simulink model "MIL_ASW"  (R2019b)
settings: Solver=FixedStepDiscrete  StartTime=0.0  StopTime=2  FixedStep=0.001  RelTol=1e-3  EnableMultiTasking=on
model workspace (MAT data in the model file):
  AccPedlCanVal : Simulink.Signal (value not decoded)
  AccPedlVal : Simulink.Signal (value not decoded)
  BrkPedlCanVal : Simulink.Signal (value not decoded)
  BrkPedlVal : Simulink.Signal (value not decoded)
  Cal1 : Simulink.Parameter (value not decoded)
  Cal10 : Simulink.Parameter (value not decoded)
  Cal11 : Simulink.Parameter (value not decoded)
  Cal12 : Simulink.Parameter (value not decoded)
  Cal2 : Simulink.Parameter (value not decoded)
  Cal3 : Simulink.Parameter (value not decoded)
  Cal4 : Simulink.Parameter (value not decoded)
  Cal5 : Simulink.Parameter (value not decoded)
  Cal6 : Simulink.Parameter (value not decoded)
  Cal7 : Simulink.Parameter (value not decoded)
  Cal8 : Simulink.Parameter (value not decoded)
  Cal9 : Simulink.Parameter (value not decoded)
  Clu1Act : Simulink.Signal (value not decoded)
  Clu1PTar : Simulink.Signal (value not decoded)
  Clu1Req : Simulink.Signal (value not decoded)
  Clu1TqTar : Simulink.Signal (value not decoded)
  Clu2Act : Simulink.Signal (value not decoded)
  Clu2PTar : Simulink.Signal (value not decoded)
  Clu2Req : Simulink.Signal (value not decoded)
  Clu2TqTar : Simulink.Signal (value not decoded)
  CluKissPtPLnch : Simulink.Parameter (value not decoded)
  CluOilTRawVal : Simulink.Signal (value not decoded)
  CluOilTVal : Simulink.Signal (value not decoded)
  CluOpenTqRatMax : Simulink.Parameter (value not decoded)
  CluPMap : Simulink.Parameter (value not decoded)
  CluPMax : Simulink.Parameter (value not decoded)
  CluPMaxGear1 : Simulink.Parameter (value not decoded)
  CluPMaxGear2 : Simulink.Parameter (value not decoded)
  CluPMaxGear3 : Simulink.Parameter (value not decoded)
  CluPMaxGear4 : Simulink.Parameter (value not decoded)
  CluPMaxGear5 : Simulink.Parameter (value not decoded)
  CluPMaxGear6 : Simulink.Parameter (value not decoded)
  CluPMaxGearR : Simulink.Parameter (value not decoded)
  CluPMin : Simulink.Parameter (value not decoded)
  CluPosnMax : Simulink.Parameter (value not decoded)
  CluSoln1IRawVal : Simulink.Signal (value not decoded)
  CluSoln1IReq : Simulink.Signal (value not decoded)
  CluSoln1IReqFlg : Simulink.Signal (value not decoded)
  CluSoln1IVal : Simulink.Signal (value not decoded)
  CluSoln1LineI : Simulink.Parameter (value not decoded)
  CluSoln1LineP : Simulink.Parameter (value not decoded)
  CluSoln1Pwm : Simulink.Signal (value not decoded)
  CluSoln2IRawVal : Simulink.Signal (value not decoded)
  CluSoln2IReq : Simulink.Signal (value not decoded)
  CluSoln2IReqFlg : Simulink.Signal (value not decoded)
  CluSoln2IVal : Simulink.Signal (value not decoded)
  CluSoln2LineI : Simulink.Parameter (value not decoded)
  CluSoln2LineP : Simulink.Parameter (value not decoded)
  CluSoln2Pwm : Simulink.Signal (value not decoded)
  CluTqMap : Simulink.Parameter (value not decoded)
  CrnkSpdRawVal : Simulink.Signal (value not decoded)
  CrnkSpdVal : Simulink.Signal (value not decoded)
  Drive_Intensity_Fuzzy : object (value not decoded)
  DrvIntenFzzy : Simulink.LookupTable (value not decoded)
  EngNIdle : Simulink.Parameter (value not decoded)
  EngNIdleMin : Simulink.Parameter (value not decoded)
  EngSpdCanVal : Simulink.Signal (value not decoded)
  EngThrCanVal : Simulink.Signal (value not decoded)
  EngTqAdd : Simulink.Parameter (value not decoded)
  EngTqCanVal : Simulink.Signal (value not decoded)
  EngTqIntvFlg : Simulink.Signal (value not decoded)
  EngTqIntvRat : Simulink.Signal (value not decoded)
  EngTqMapExtChartc : Simulink.Parameter (value not decoded)
  EngTqMapSpdIndx : Simulink.Parameter (value not decoded)
  EngTqMapThrtIndx : Simulink.Parameter (value not decoded)
  EngTqMapTqMax : Simulink.Parameter (value not decoded)
  EngTqMaxNorm : Simulink.Parameter (value not decoded)
  EngTqRef : Simulink.Parameter (value not decoded)
  EvenCluPRawVal : Simulink.Signal (value not decoded)
  EvenCluPVal : Simulink.Signal (value not decoded)
  EvenInpSpdRawVal : Simulink.Signal (value not decoded)
  EvenInpSpdVal : Simulink.Signal (value not decoded)
  FcnCallTime : Simulink.Parameter (value not decoded)
  FinalRat : Simulink.Parameter (value not decoded)
  Fork1A : Simulink.Parameter (value not decoded)
  Fork1Act : Simulink.Signal (value not decoded)
  Fork1B : Simulink.Parameter (value not decoded)
  Fork1DeltaSpdTar : Simulink.Parameter (value not decoded)
  Fork1MaxSpd1A : Simulink.Parameter (value not decoded)
  Fork1MaxSpd1B : Simulink.Parameter (value not decoded)
  Fork1MaxSpd2A : Simulink.Parameter (value not decoded)
  Fork1MaxSpd2B : Simulink.Parameter (value not decoded)
  Fork1PosnA : Simulink.Parameter (value not decoded)
  Fork1PosnB : Simulink.Parameter (value not decoded)
  Fork1PosnMaxSpd1A : Simulink.Parameter (value not decoded)
  Fork1PosnMaxSpd1B : Simulink.Parameter (value not decoded)
  Fork1PosnMaxSpd2A : Simulink.Parameter (value not decoded)
  Fork1PosnMaxSpd2B : Simulink.Parameter (value not decoded)
  Fork1PosnNeut : Simulink.Parameter (value not decoded)
  Fork1PosnNeutA : Simulink.Parameter (value not decoded)
  Fork1PosnNeutB : Simulink.Parameter (value not decoded)
  Fork1PosnRawVal : Simulink.Signal (value not decoded)
  Fork1PosnSyncA : Simulink.Parameter (value not decoded)
  Fork1PosnSyncB : Simulink.Parameter (value not decoded)
  Fork1PosnVal : Simulink.Signal (value not decoded)
  Fork1SyncTar : Simulink.Parameter (value not decoded)
  Fork2A : Simulink.Parameter (value not decoded)
  Fork2Act : Simulink.Signal (value not decoded)
  Fork2B : Simulink.Parameter (value not decoded)
  Fork2DeltaSpdTar : Simulink.Parameter (value not decoded)
  Fork2MaxSpd1A : Simulink.Parameter (value not decoded)
  Fork2MaxSpd1B : Simulink.Parameter (value not decoded)
  Fork2MaxSpd2A : Simulink.Parameter (value not decoded)
  Fork2MaxSpd2B : Simulink.Parameter (value not decoded)
  Fork2PosnA : Simulink.Parameter (value not decoded)
  Fork2PosnB : Simulink.Parameter (value not decoded)
  Fork2PosnMaxSpd1A : Simulink.Parameter (value not decoded)
  Fork2PosnMaxSpd1B : Simulink.Parameter (value not decoded)
  Fork2PosnMaxSpd2A : Simulink.Parameter (value not decoded)
  Fork2PosnMaxSpd2B : Simulink.Parameter (value not decoded)
  Fork2PosnNeut : Simulink.Parameter (value not decoded)
  Fork2PosnNeutA : Simulink.Parameter (value not decoded)
  Fork2PosnNeutB : Simulink.Parameter (value not decoded)
  Fork2PosnRawVal : Simulink.Signal (value not decoded)
  Fork2PosnSyncA : Simulink.Parameter (value not decoded)
  Fork2PosnSyncB : Simulink.Parameter (value not decoded)
  Fork2PosnVal : Simulink.Signal (value not decoded)
  Fork2SyncTar : Simulink.Parameter (value not decoded)
  Fork3A : Simulink.Parameter (value not decoded)
  Fork3Act : Simulink.Signal (value not decoded)
  Fork3B : Simulink.Parameter (value not decoded)
  Fork3DeltaSpdTar : Simulink.Parameter (value not decoded)
  Fork3MaxSpd1A : Simulink.Parameter (value not decoded)
  Fork3MaxSpd1B : Simulink.Parameter (value not decoded)
  Fork3MaxSpd2A : Simulink.Parameter (value not decoded)
  Fork3MaxSpd2B : Simulink.Parameter (value not decoded)
  Fork3PosnA : Simulink.Parameter (value not decoded)
  Fork3PosnB : Simulink.Parameter (value not decoded)
  Fork3PosnMaxSpd1A : Simulink.Parameter (value not decoded)
  Fork3PosnMaxSpd1B : Simulink.Parameter (value not decoded)
  Fork3PosnMaxSpd2A : Simulink.Parameter (value not decoded)
  Fork3PosnMaxSpd2B : Simulink.Parameter (value not decoded)
  Fork3PosnNeut : Simulink.Parameter (value not decoded)
  Fork3PosnNeutA : Simulink.Parameter (value not decoded)
  Fork3PosnNeutB : Simulink.Parameter (value not decoded)
  Fork3PosnRawVal : Simulink.Signal (value not decoded)
  Fork3PosnSyncA : Simulink.Parameter (value not decoded)
  Fork3PosnSyncB : Simulink.Parameter (value not decoded)
  Fork3PosnVal : Simulink.Signal (value not decoded)
  Fork3SyncTar : Simulink.Parameter (value not decoded)
  Fork4A : Simulink.Parameter (value not decoded)
  Fork4Act : Simulink.Signal (value not decoded)
  Fork4B : Simulink.Parameter (value not decoded)
  Fork4DeltaSpdTar : Simulink.Parameter (value not decoded)
  Fork4MaxSpd1A : Simulink.Parameter (value not decoded)
  Fork4MaxSpd1B : Simulink.Parameter (value not decoded)
  Fork4MaxSpd2A : Simulink.Parameter (value not decoded)
  Fork4MaxSpd2B : Simulink.Parameter (value not decoded)
  Fork4PosnA : Simulink.Parameter (value not decoded)
  Fork4PosnB : Simulink.Parameter (value not decoded)
  Fork4PosnMaxSpd1A : Simulink.Parameter (value not decoded)
  Fork4PosnMaxSpd1B : Simulink.Parameter (value not decoded)
  Fork4PosnMaxSpd2A : Simulink.Parameter (value not decoded)
  Fork4PosnMaxSpd2B : Simulink.Parameter (value not decoded)
  Fork4PosnNeut : Simulink.Parameter (value not decoded)
  Fork4PosnNeutA : Simulink.Parameter (value not decoded)
  Fork4PosnNeutB : Simulink.Parameter (value not decoded)
  Fork4PosnRawVal : Simulink.Signal (value not decoded)
  Fork4PosnSyncA : Simulink.Parameter (value not decoded)
  Fork4PosnSyncB : Simulink.Parameter (value not decoded)
  Fork4PosnVal : Simulink.Signal (value not decoded)
  Fork4SyncTar : Simulink.Parameter (value not decoded)
  FrntWhlRd : Simulink.Parameter (value not decoded)
  GearIdx : Simulink.Parameter (value not decoded)
  GearMax : Simulink.Parameter (value not decoded)
  GearRat : Simulink.Parameter (value not decoded)
  Launch_Engage_Fuzzy : object (value not decoded)
  LnchEngmtFzzy : Simulink.LookupTable (value not decoded)
  LubeSolnIRawVal : Simulink.Signal (value not decoded)
  LubeSolnIReq : Simulink.Signal (value not decoded)
  LubeSolnIVal : Simulink.Signal (value not decoded)
  LubeSolnLineI : Simulink.Parameter (value not decoded)
  LubeSolnLineP : Simulink.Parameter (value not decoded)
  LubeSolnPwm : Simulink.Signal (value not decoded)
  MaiLineSolnIRawVal : Simulink.Signal (value not decoded)
  MaiLineSolnIReq : Simulink.Signal (value not decoded)
  MaiLineSolnIVal : Simulink.Signal (value not decoded)
  MaiLineSolnLineI : Simulink.Parameter (value not decoded)
  MaiLineSolnLineP : Simulink.Parameter (value not decoded)
  MaiLineSolnPwm : Simulink.Signal (value not decoded)
  OddCluPRawVal : Simulink.Signal (value not decoded)
  OddCluPVal : Simulink.Signal (value not decoded)
  OddInpSpdRawVal : Simulink.Signal (value not decoded)
  OddInpSpdVal : Simulink.Signal (value not decoded)
  OutpSpdRawVal : Simulink.Signal (value not decoded)
  OutpSpdVal : Simulink.Signal (value not decoded)
  PsnsrLineP : Simulink.Parameter (value not decoded)
  PsnsrLineV : Simulink.Parameter (value not decoded)
  SftLvrCanVal : Simulink.Signal (value not decoded)
  SftLvrCfm : Simulink.Signal (value not decoded)
  SftLvrVal : Simulink.Signal (value not decoded)
  Shaft1GearAct : Simulink.Signal (value not decoded)
  Shaft1GearReq : Simulink.Signal (value not decoded)
  Shaft2GearAct : Simulink.Signal (value not decoded)
  Shaft2GearReq : Simulink.Signal (value not decoded)
  ShiftMux1SwtReq : Simulink.Signal (value not decoded)
  ShiftMux2SwtReq : Simulink.Signal (value not decoded)
  ShiftSdlEcoDwnSeln : Simulink.Parameter (value not decoded)
  ShiftSdlEcoDwnShift : Simulink.Parameter (value not decoded)
  ShiftSdlEcoUpSeln : Simulink.Parameter (value not decoded)
  ShiftSdlEcoUpShift : Simulink.Parameter (value not decoded)
  ShiftSdlPwrDwnSeln : Simulink.Parameter (value not decoded)
  ShiftSdlPwrDwnShift : Simulink.Parameter (value not decoded)
  ShiftSdlPwrUpSeln : Simulink.Parameter (value not decoded)
  ShiftSdlPwrUpShift : Simulink.Parameter (value not decoded)
  ShiftSdlSACDwnSeln : Simulink.Parameter (value not decoded)
  ShiftSdlSACDwnShift : Simulink.Parameter (value not decoded)
  ShiftSdlSACUpSeln : Simulink.Parameter (value not decoded)
  ShiftSdlSACUpShift : Simulink.Parameter (value not decoded)
  ShiftSdlThrPedlIdx : Simulink.Parameter (value not decoded)
  ShiftSoln1IRawVal : Simulink.Signal (value not decoded)
  ShiftSoln1IReq : Simulink.Signal (value not decoded)
  ShiftSoln1IVal : Simulink.Signal (value not decoded)
  ShiftSoln1LineI : Simulink.Parameter (value not decoded)
  ShiftSoln1LineP : Simulink.Parameter (value not decoded)
  ShiftSoln1Pwm : Simulink.Signal (value not decoded)
  ShiftSoln2IRawVal : Simulink.Signal (value not decoded)
  ShiftSoln2IReq : Simulink.Signal (value not decoded)
  ShiftSoln2IVal : Simulink.Signal (value not decoded)
  ShiftSoln2LineI : Simulink.Parameter (value not decoded)
  ShiftSoln2LineP : Simulink.Parameter (value not decoded)
  ShiftSoln2Pwm : Simulink.Signal (value not decoded)
  SolnOutpTRawVal : Simulink.Signal (value not decoded)
  SolnOutpTVal : Simulink.Signal (value not decoded)
  TSnsr1LineR : Simulink.Parameter (value not decoded)
  TSnsr2LineR : Simulink.Parameter (value not decoded)
  TrsmNrGearAct : Simulink.Signal (value not decoded)
  TrsmNrGearReq : Simulink.Signal (value not decoded)
  TrsmNrPreGearAct : Simulink.Signal (value not decoded)
  TrsmNrPreGearReq : Simulink.Signal (value not decoded)
  Tsnsr1LineT : Simulink.Parameter (value not decoded)
  Tsnsr2LineT : Simulink.Parameter (value not decoded)
  VehSpdCanVal : Simulink.Signal (value not decoded)
  VehSpdTrsmEstimd : Simulink.Signal (value not decoded)
  VehSpdVal : Simulink.Signal (value not decoded)
  VlvBodyTRawVal : Simulink.Signal (value not decoded)
  VlvBodyTVal : Simulink.Signal (value not decoded)
symbols that are objects in the model workspace (value not decoded): CluPMap, CluSoln1LineI, CluSoln1LineP, CluSoln2LineI, CluSoln2LineP, CluTqMap, EngNIdle, EngNIdleMin, EngTqMapThrtIndx, EngTqMapTqMax, EngTqMaxNorm, FcnCallTime, FinalRat, Fork1A, Fork1B, Fork1DeltaSpdTar, Fork1PosnA, Fork1PosnB, Fork1PosnMaxSpd1A, Fork1PosnMaxSpd1B, Fork1PosnMaxSpd2A, Fork1PosnMaxSpd2B, Fork1PosnNeut, Fork1PosnNeutA, Fork1PosnNeutB, Fork1PosnSyncA, Fork1PosnSyncB, Fork1SyncTar, Fork2A, Fork2B, Fork2DeltaSpdTar, Fork2PosnA, Fork2PosnB, Fork2PosnMaxSpd1A, Fork2PosnMaxSpd1B, Fork2PosnMaxSpd2A, Fork2PosnMaxSpd2B, Fork2PosnNeut, Fork2PosnNeutA, Fork2PosnNeutB, Fork2PosnSyncA, Fork2PosnSyncB, Fork2SyncTar, Fork3A, Fork3B, Fork3DeltaSpdTar, Fork3PosnA, Fork3PosnB, Fork3PosnMaxSpd1A, Fork3PosnMaxSpd1B, Fork3PosnMaxSpd2A, Fork3PosnMaxSpd2B, Fork3PosnNeut, Fork3PosnNeutA, Fork3PosnNeutB, Fork3PosnSyncA, Fork3PosnSyncB, Fork3SyncTar, Fork4A, Fork4B
undefined symbols (not defined in the file or in its folder): in1, out1
libraries: simulink x44, fuzblock x3
(part 10 of 10)

== stateflow chart MIL_ASW/Application_Software_SHAW/ASW_ShaftAccessControl/Shift lever match to gear/Shift lever confirm logic ==
  state P
    en:
    SftLvrCfm= uint8(0);
  state R
    en:
    SftLvrCfm= uint8(1);
  state N
    en:
    SftLvrCfm= uint8(2);
  state D
    en:
    SftLvrCfm= uint8(3);
  state W
    en:
    SftLvrCfm= uint8(4);
  state wait
  (junction 39) -> (junction 41)
  (junction 41) -> (junction 44) [order 2]
  (junction 44) -> (junction 47) [order 2]
  (junction 47) -> (junction 50) [order 2]
  (junction 50) -> (junction 53) [order 2]
  wait -> (junction 39)
  (junction 41) -> P [order 1] : [ShiftLvrRx==uint8(0)&&...
      | GearRx==uint8(0)&&...
      | PreGearRx==uint8(0)]
  (junction 44) -> R [order 1] : [ShiftLvrRx==uint8(1)&&...
      | PreGearRx==uint8(7)]
  (junction 47) -> N [order 1] : [ShiftLvrRx==uint8(2)&&...
      | GearRx==uint8(0)&&...
      | PreGearRx==uint8(0)]
  (junction 50) -> D [order 1] : [ShiftLvrRx==uint8(3)&&...
      | GearRx<uint8(7)&&...
      | (PreGearRx>uint8(0)&&...
      | PreGearRx<uint8(7))]
  (junction 53) -> W : [ShiftLvrRx==uint8(4)&&...
      | GearRx<uint8(7)&&...
      | (PreGearRx>uint8(0)&&...
      | PreGearRx<uint8(7))]
  (default) -> wait
  (junction 21) -> wait
  P -> (junction 12) : [ShiftLvrRx~=uint8(0)]
  R -> (junction 27) : [ShiftLvrRx~=uint8(1)]
  N -> (junction 29) : [ShiftLvrRx~=uint8(2)]
  D -> (junction 32) : [ShiftLvrRx~=uint8(3)]
  W -> (junction 35) : [ShiftLvrRx~=uint8(4)]
  (junction 12) -> (junction 21)
  (junction 27) -> (junction 12)
  (junction 29) -> (junction 27)
  (junction 32) -> (junction 29)
  (junction 35) -> (junction 32)
  data: ShiftLvrRx input uint8 size=1; GearRx input uint8 size=1; PreGearRx input uint8 size=1; SftLvrCfm output uint8 size=1

== stateflow chart MIL_ASW/Application_Software_SHAW/ASW_ShaftControl/Even Part ==
  state initailize
    en:
    Shaft2GearAct=0;
  state wait
  state DisengageErrorCheck
    en:ErrCntFork++;
  state Disengage2ErrorCheck
    en:ErrCntFork++;
  state Fork2_Disengage
    en:Fork2Req=0;
    Cntr=10;
    du:Cntr--;
  state Fork4_Disengage
    en:Fork4Req=0;
    Cntr=10;
    du:Cntr--;
  state Engage2ErrorCheck1
    en:ErrCntFork++;
  state DisengageErrorCheck1
    en:ErrCntFork++;
  state Fork4_Disengage1
    en:Fork4Req=0;
    Cntr=10;
    du:Cntr--;
  state GearPositionerFork2
    en:Fork2Req=Shaft2GearReqLoc;
    Cntr=10;
    du:Cntr--;
  state Disengage2ErrorCheck1
    en:ErrCntFork++;
  state Engage2ErrorCheck
    en:ErrCntFork++;
  state GearPositionerFork4
    en:Fork4Req=Shaft2GearReqLoc;
    Cntr=10;
    du:Cntr--;
  state Fork2_Disengage1
    en:Fork2Req=0;
    Cntr=10;
    du:Cntr--;
  state ErrorOutput
  state ShiftSuccess
    en:Shaft2GearAct=Shaft2GearReqLoc;
    Shaft2GearErr=0;
  (default) -> initailize
  initailize -> wait
  (junction 307) -> wait
  (junction 453) -> wait
  (junction 314) -> (junction 307)
  ErrorOutput -> (junction 453)
  wait -> (junction 501) [order 1] : [Shaft2GearReq!=Shaft2GearAct]
  wait -> (junction 503) [order 2] : [Shaft2GearReq==0&&...
      | (Fork2Act!=0||Fork4Act!=0)]
  wait -> (junction 506) [order 3] : [Shaft2GearReq!=0&&...
      | (Shaft2GearReq!=Fork2Act&&Shaft2GearReq!=Fork4Act)]
  (junction 371) -> (junction 449)
  (junction 449) -> (junction 370)
  DisengageErrorCheck -> (junction 371) [order 2] : {Shaft2GearErr=1;}
  Disengage2ErrorCheck -> (junction 449) [order 2] : {Shaft2GearErr=2;}
  (junction 370) -> (junction 475)
  Fork4_Disengage -> Disengage2ErrorCheck [order 2] : [Cntr<=0]
  Disengage2ErrorCheck -> Fork4_Disengage [order 1] : [ErrCntFork<4]
  Fork2_Disengage -> DisengageErrorCheck [order 2] : [Cntr<=0]
  DisengageErrorCheck -> Fork2_Disengage [order 1] : [ErrCntFork<4]
  (junction 501) -> (junction 503)
  (junction 506) -> (junction 503)
  (junction 503) -> (junction 451) : {Shaft2GearReqLoc=Shaft2GearReq;}
  Fork2_Disengage -> Fork4_Disengage [order 1] : [Fork2Act==0]
      | {ErrCntFork=0;}
  (junction 451) -> Fork2_Disengage [order 1] : [Shaft2GearReqLoc==0]
      | {ErrCntFork=0;}
  Fork4_Disengage -> (junction 456) [order 1] : [Fork4Act==0]
  (junction 451) -> (junction 360) [order 2]
  (junction 456) -> (junction 473)
  (junction 468) -> (junction 469)
  (junction 469) -> (junction 475)
  DisengageErrorCheck1 -> (junction 468) [order 2] : {Shaft2GearErr=3;}
  Engage2ErrorCheck1 -> (junction 469) [order 2] : {Shaft2GearErr=4;}
  (junction 475) -> (junction 490)
  Fork4_Disengage1 -> DisengageErrorCheck1 [order 2] : [Cntr<=0]
  DisengageErrorCheck1 -> Fork4_Disengage1 [order 1] : [ErrCntFork<4]
  GearPositionerFork2 -> Engage2ErrorCheck1 [order 2] : [Cntr<=0]
  Engage2ErrorCheck1 -> GearPositionerFork2 [order 1] : [ErrCntFork<4]
  Fork4_Disengage1 -> GearPositionerFork2 [order 1] : [Fork4Act==0]
      | {ErrCntFork=0;}
  (junction 360) -> Fork4_Disengage1 [order 1] : [Shaft2GearReqLoc==Fork2A||...
      | Shaft2GearReqLoc==Fork2B]
      | {ErrCntFork=0;}
  GearPositionerFork2 -> (junction 473) [order 1] : [Fork2Act==Shaft2GearReqLoc]
  (junction 360) -> (junction 190) [order 2]
  (junction 473) -> (junction 387)
  (junction 488) -> (junction 489)
  (junction 489) -> (junction 490)
  Disengage2ErrorCheck1 -> (junction 488) [order 2] : {Shaft2GearErr=5;}
  Engage2ErrorCheck -> (junction 489) [order 2] : {Shaft2GearErr=6;}
  (junction 490) -> (junction 494)
  GearPositionerFork4 -> Engage2ErrorCheck [order 2] : [Cntr<=0]
  Engage2ErrorCheck -> GearPositionerFork4 [order 1] : [ErrCntFork<4]
  Fork2_Disengage1 -> Disengage2ErrorCheck1 [order 2] : [Cntr<=0]
  Disengage2ErrorCheck1 -> Fork2_Disengage1 [order 1] : [ErrCntFork<4]
  Fork2_Disengage1 -> GearPositionerFork4 [order 1] : [Fork2Act==0]
      | {ErrCntFork=0;}
  (junction 190) -> Fork2_Disengage1 [order 1] : [Shaft2GearReqLoc==Fork4A||...
      | Shaft2GearReqLoc==Fork4B]
      | {ErrCntFork=0;}
  GearPositionerFork4 -> (junction 387) [order 1] : [Fork4Act==Shaft2GearReqLoc]
  (junction 190) -> (junction 492) [order 2]
  (junction 387) -> (junction 496)
  (junction 492) -> (junction 494) : {Shaft2GearErr=7;}
  (junction 494) -> ErrorOutput
  ShiftSuccess -> (junction 314)
  (junction 496) -> ShiftSuccess
  data: Fork2Act input uint8; Fork4Act input uint8; Shaft2GearReq input uint8; Fork2Req output uint8; Fork4Req output uint8; Shaft2GearAct output uint8; Shaft2GearErr output uint8; Shaft2GearReqLoc local uint8; Cntr local uint8; ErrCntFork local uint8; Fork2A parameter uint8; Fork2B parameter uint8; Fork4A parameter uint8; Fork4B parameter uint8

== stateflow chart MIL_ASW/Application_Software_SHAW/ASW_ShaftControl/Odd Part ==
  state initailize
    en:
    Shaft1GearAct=0;
  state wait
  state DisengageErrorCheck
    en:ErrCntFork++;
  state Disengage2ErrorCheck
    en:ErrCntFork++;
  state Fork1_Disengage
    en:Fork1Req=0;
    Cntr=10;
    du:Cntr--;
  state Fork3_Disengage
    en:Fork3Req=0;
    Cntr=10;
    du:Cntr--;
  state Engage2ErrorCheck1
    en:ErrCntFork++;
  state DisengageErrorCheck1
    en:ErrCntFork++;
  state Fork3_Disengage1
    en:Fork3Req=0;
    Cntr=10;
    du:Cntr--;
  state GearPositionerFork1
    en:Fork1Req=Shaft1GearReqLoc;
    Cntr=10;
    du:Cntr--;
  state Disengage2ErrorCheck1
    en:ErrCntFork++;
  state Engage2ErrorCheck
    en:ErrCntFork++;
  state GearPositionerFork3
    en:Fork3Req=Shaft1GearReqLoc;
    Cntr=10;
    du:Cntr--;
  state Fork1_Disengage1
    en:Fork1Req=0;
    Cntr=10;
    du:Cntr--;
  state ErrorOutput
  state ShiftSuccess
    en:Shaft1GearAct=Shaft1GearReqLoc;
    Shaft1GearErr=0;
  (default) -> initailize
  initailize -> wait
  (junction 307) -> wait
  (junction 453) -> wait
  (junction 314) -> (junction 307)
  ErrorOutput -> (junction 453)
  wait -> (junction 501) [order 1] : [Shaft1GearReq!=Shaft1GearAct]
  wait -> (junction 503) [order 2] : [Shaft1GearReq==0&&...
      | (Fork1Act!=0||Fork3Act!=0)]
  wait -> (junction 506) [order 3] : [Shaft1GearReq!=0&&...
      | (Shaft1GearReq!=Fork1Act&&Shaft1GearReq!=Fork3Act)]
  (junction 371) -> (junction 449)
  (junction 449) -> (junction 370)
  DisengageErrorCheck -> (junction 371) [order 2] : {Shaft1GearErr=1;}
  Disengage2ErrorCheck -> (junction 449) [order 2] : {Shaft1GearErr=2;}
  (junction 370) -> (junction 475)
  Fork3_Disengage -> Disengage2ErrorCheck [order 2] : [Cntr<=0]
  Disengage2ErrorCheck -> Fork3_Disengage [order 1] : [ErrCntFork<4]
  Fork1_Disengage -> DisengageErrorCheck [order 2] : [Cntr<=0]
  DisengageErrorCheck -> Fork1_Disengage [order 1] : [ErrCntFork<4]
  (junction 501) -> (junction 503)
  (junction 506) -> (junction 503)
  (junction 503) -> (junction 451) : {Shaft1GearReqLoc=Shaft1GearReq;}
  Fork1_Disengage -> Fork3_Disengage [order 1] : [Fork1Act==0]
      | {ErrCntFork=0;}
  (junction 451) -> Fork1_Disengage [order 1] : [Shaft1GearReqLoc==0]
      | {ErrCntFork=0;}
  Fork3_Disengage -> (junction 456) [order 1] : [Fork3Act==0]
  (junction 451) -> (junction 360) [order 2]
  (junction 456) -> (junction 473)
  (junction 468) -> (junction 469)
  (junction 469) -> (junction 475)
  DisengageErrorCheck1 -> (junction 468) [order 2] : {Shaft1GearErr=3;}
  Engage2ErrorCheck1 -> (junction 469) [order 2] : {Shaft1GearErr=4;}
  (junction 475) -> (junction 490)
  Fork3_Disengage1 -> DisengageErrorCheck1 [order 2] : [Cntr<=0]
  DisengageErrorCheck1 -> Fork3_Disengage1 [order 1] : [ErrCntFork<4]
  GearPositionerFork1 -> Engage2ErrorCheck1 [order 2] : [Cntr<=0]
  Engage2ErrorCheck1 -> GearPositionerFork1 [order 1] : [ErrCntFork<4]
  Fork3_Disengage1 -> GearPositionerFork1 [order 1] : [Fork3Act==0]
      | {ErrCntFork=0;}
  (junction 360) -> Fork3_Disengage1 [order 1] : [Shaft1GearReqLoc==Fork1A||...
      | Shaft1GearReqLoc==Fork1B]
      | {ErrCntFork=0;}
  GearPositionerFork1 -> (junction 473) [order 1] : [Fork1Act==Shaft1GearReqLoc]
  (junction 360) -> (junction 190) [order 2]
  (junction 473) -> (junction 387)
  (junction 488) -> (junction 489)
  (junction 489) -> (junction 490)
  Disengage2ErrorCheck1 -> (junction 488) [order 2] : {Shaft1GearErr=5;}
  Engage2ErrorCheck -> (junction 489) [order 2] : {Shaft1GearErr=6;}
  (junction 490) -> (junction 494)
  GearPositionerFork3 -> Engage2ErrorCheck [order 2] : [Cntr<=0]
  Engage2ErrorCheck -> GearPositionerFork3 [order 1] : [ErrCntFork<4]
  Fork1_Disengage1 -> Disengage2ErrorCheck1 [order 2] : [Cntr<=0]
  Disengage2ErrorCheck1 -> Fork1_Disengage1 [order 1] : [ErrCntFork<4]
  Fork1_Disengage1 -> GearPositionerFork3 [order 1] : [Fork1Act==0]
      | {ErrCntFork=0;}
  (junction 190) -> Fork1_Disengage1 [order 1] : [Shaft1GearReqLoc==Fork3A||...
      | Shaft1GearReqLoc==Fork3B]
      | {ErrCntFork=0;}
  GearPositionerFork3 -> (junction 387) [order 1] : [Fork3Act==Shaft1GearReqLoc]
  (junction 190) -> (junction 492) [order 2]
  (junction 387) -> (junction 496)
  (junction 492) -> (junction 494) : {Shaft1GearErr=7;}
  (junction 494) -> ErrorOutput
  ShiftSuccess -> (junction 314)
  (junction 496) -> ShiftSuccess
  data: Fork1Act input uint8; Fork3Act input uint8; Shaft1GearReq input uint8; Fork1Req output uint8; Fork3Req output uint8; Shaft1GearAct output uint8; Shaft1GearErr output uint8; Shaft1GearReqLoc local uint8; Cntr local uint8; ErrCntFork local uint8; Fork1A parameter uint8; Fork1B parameter uint8; Fork3A parameter uint8; Fork3B parameter uint8
